simulink model "Hydraulic_Hybrid_direct"  (R2012b)
settings: Solver=ode4  StartTime=0.0  StopTime=length(speed_U)-1  FixedStep=t_samp_d  RelTol=1e-3
values from neighbouring files (symbols this model uses):
  Af = param_Af(i)    [parametric_analysis.m]    (also in settings.m = 2)
  alpha = 14.7    [settings.m]
  Cd = param_Cd(i)    [parametric_analysis.m]    (also in settings.m = 0.3)
  CHARGE_p = 0.7    [settings.m]
  eps_p = param_eps_p(i)    [parametric_analysis.m]    (also in settings.m = 3)
  eta_mech = param_eta_mech(i)    [parametric_analysis.m]    (also in settings.m = 0.8)
  f = param_f(i)    [parametric_analysis.m]    (also in settings.m = 0.015)
  gear_ratios = param_gear_ratios(i,:)    [parametric_analysis.m]    (also in settings.m = [3.6 2.1 1.4 1 0.8])
  k = 1.4    [settings.m]
  Kd = param_Kd(i)    [parametric_analysis.m]    (also in settings.m = 0.1)
  m = param_m(i)    [parametric_analysis.m]    (also in settings.m = 1200)
  n_ICE_etamax = param_n_ICE_etamax(i)    [parametric_analysis.m]    (also in settings.m = 2500)
  p_ACC_0 = param_p_ACC_0(i)    [parametric_analysis.m]    (also in settings.m = 24000000)
  p_ACC_MAX = param_p_ACC_MAX(i)    [parametric_analysis.m]    (also in settings.m = 35000000)
  p_ACC_min = param_p_ACC_min(i)    [parametric_analysis.m]    (also in settings.m = 13000000)
  p_SERB_0 = param_p_SERB_0(i)    [parametric_analysis.m]    (also in settings.m = 760000)
  p_SERB_MAX = param_p_SERB_MAX(i)    [parametric_analysis.m]    (also in settings.m = 1800000)
  p_SERB_min = param_p_SERB_min(i)    [parametric_analysis.m]    (also in settings.m = 600000)
  r_ROT = param_r_ROT(i)    [parametric_analysis.m]    (also in settings.m = 0.26)
  rho_air = 1.2    [settings.m]
  rho_fuel = 720    [settings.m]
  slope = [0 0 0 0 0 0 0 0 0 0 0 0 ... (1370 elements, 1370x1)]    [cycles.mat]
  speed_H = [0 0 0 3.22 7.889 13.041 18.193 23.345 27.853 31.556 35.098 38.64 ... (1370 elements, 1370x1)]    [cycles.mat]
  speed_U = [0 0 0 0 0 0 0 0 0 0 0 0 ... (1370 elements, 1370x1)]    [cycles.mat]
  T_brake_MAX = 200    [settings.m]
  T_n_MAX = param_T_n_MAX(i)    [parametric_analysis.m]    (also in settings.m = 60)
  T_n_min = param_T_n_min(i)    [parametric_analysis.m]    (also in settings.m = 40)
  t_react = param_t_react(i)    [parametric_analysis.m]    (also in settings.m = 0.1)
  t_samp = 1    [settings.m]
  t_samp_d = 1/5    (= 0.2)    [settings.m]
  tau = param_tau(i)    [parametric_analysis.m]    (also in settings.m = 0.1)
  torque_curve = param_torque_curve(i,:)    [parametric_analysis.m]    (also in settings.m = [n_ICE_min;(T_MAX-T_n_min)/(n_TM_min-n_ICE_min);n_TM_min;T_M)
  V_ACC_0 = param_V_ACC_0(i)    [parametric_analysis.m]    (also in settings.m = 0.0323)
  V_ICE = param_V_ICE(i)    [parametric_analysis.m]    (also in settings.m = 0.0014)
  V_PM = 45*10^(-6)    (= 4.5e-05)    [settings.m]
  V_SERB_0 = param_V_SERB_0(i)    [parametric_analysis.m]    (also in settings.m = 0.0423)
  wind_speed = [0 0 0 0 0 0 0 0 0 0 0 0 ... (1370 elements, 1370x1)]    [cycles.mat]
settings Model: Creator=MEGA  LastModifiedBy=MEGA

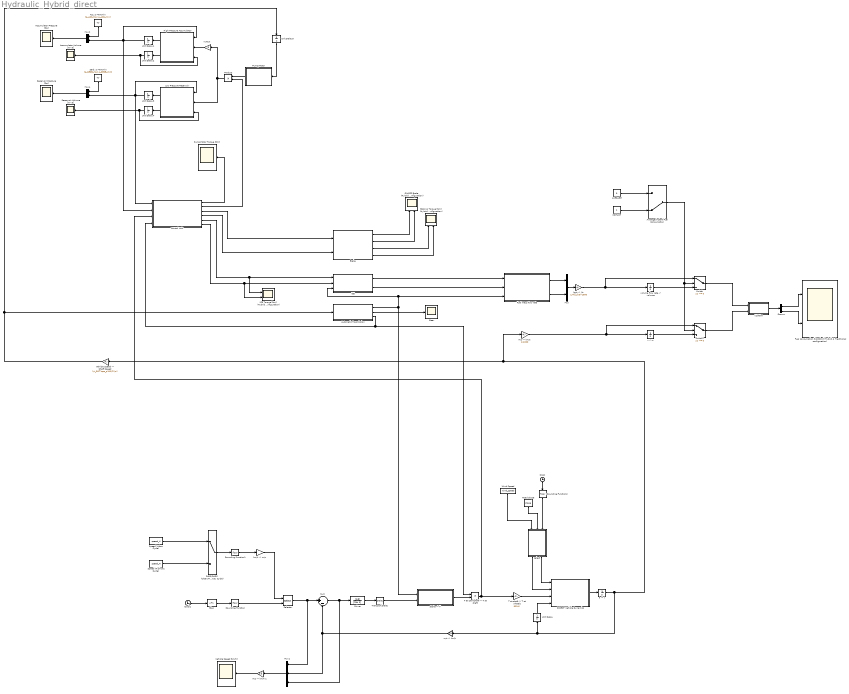
== system Hydraulic_Hybrid_direct ==
  AVERAGE : Constant  Value=0  SampleTime=t_samp_d
  Acc. p MAX/min : Constant  Value=[p_ACC_MAX p_ACC_min]  SampleTime=t_samp_d
  Accumulator Pressure [Pa] : Scope
      settings: SaveName=accum_press  SampleInput=on  SampleTime=t_samp_d
  Accumulator Volume [m^3] : Scope
      settings: SaveName=accum_vol  SampleInput=on  SampleTime=t_samp_d
  Automatic Trasmission : MATLAB Function  TreatAsAtomicUnit=on  SystemSampleTime=t_samp_d
  Average/Instant Fuel Consumption : ManualSwitch  CurrentSetting=0  SampleTime=t_samp_d
  Bias : Bias  Bias=1
  Brake : MATLAB Function  TreatAsAtomicUnit=on  SystemSampleTime=t_samp_d
  Braking Torque [Nm] (Hybrid & Traditional Configuration) : Scope  NumInputPorts=2
      settings: YMin=-5~-5  YMax=5~5  SaveName=brake_torque  DataFormat=Structure  SampleInput=on  SampleTime=t_samp_d
  Clock : Clock
  Clock1 : Clock
  Control Unit : MATLAB Function  TreatAsAtomicUnit=on  SystemSampleTime=t_samp_d
  DIRECT Vehicle Dynamics : MATLAB Function  TreatAsAtomicUnit=on  SystemSampleTime=t_samp_d
  Demux : Demux  Outputs=2
  Driver : TransferFcn  Numerator=[Kd]  Denominator=[tau 1]
  FUDS/FHDS (Urban/Highway Cycle) : ManualSwitch  SampleTime=t_samp_d
  Fuel consumption [l/100km] (Hybrid & Traditional configuration) : Scope  NumInputPorts=2
      settings: YMin=0.485~5.57  YMax=0.56~5.77  SaveName=fuel_consumption  DataFormat=Structure  SampleInput=on  SampleTime=t_samp_d
  Fuel mass flow rate : MATLAB Function  TreatAsAtomicUnit=on  SystemSampleTime=t_samp_d
  Gear : Scope
      settings: YMin=0.95  YMax=1.05  SaveName=gear  SampleInput=on  SampleTime=t_samp_d
  High Pressure Accumulator : MATLAB Function  TreatAsAtomicUnit=on  SystemSampleTime=t_samp_d
  ICE : MATLAB Function  TreatAsAtomicUnit=on  SystemSampleTime=t_samp_d
  ICE Torque [Nm] (Hybrid & Traditional Configuration) : Scope  NumInputPorts=2
      settings: YMin=-5~-5  YMax=5~5  SaveName=ICE_torque  DataFormat=Structure  SampleInput=on  SampleTime=t_samp_d
  INSTANT : Constant  SampleTime=t_samp_d
  In/Out : Gain  Gain=-1  SampleTime=t_samp_d
  Low Pressure Reservoir : MATLAB Function  TreatAsAtomicUnit=on  SystemSampleTime=t_samp_d
  Mux : Mux  Inputs=2
  Mux1 : Mux  Inputs=3
  Mux2 : Mux  Inputs=2
  Mux4 : Mux  Inputs=2
  ON/OFF Brake (Hybrid & Traditional Configuration) : Scope  NumInputPorts=2
      settings: ShowLegends=on  YMin=-5~-5  YMax=5~5  SampleInput=on  SampleTime=t_samp_d
  Product : Product  SampleTime=t_samp_d  RndMeth=Zero
  Pump/Motor : MATLAB Function  TreatAsAtomicUnit=on  SystemSampleTime=t_samp_d
  Pump/Motor Torque [Nm] : Scope
      settings: YMin=0  YMax=42.5  SaveName=hyd_torque  SampleInput=on  SampleTime=t_samp_d
  Reservoir Pressure [Pa] : Scope
      settings: SaveName=serb_press  SampleInput=on  SampleTime=t_samp_d
  Reservoir Volume [m^3] : Scope
      settings: SaveName=serb_vol  SampleInput=on  SampleTime=t_samp_d
  Road Slope : Constant  Value=slope  SampleTime=t_samp_d
  Rounding Function : Rounding  SampleTime=t_samp_d
  Rounding Function1 : Rounding  SampleTime=t_samp_d
  Rounding Function2 : Rounding  SampleTime=t_samp_d
  Selector : Selector  InputPortWidth=1370  SampleTime=t_samp_d  IndexOptions=Index vector (port)  Indices=[1 3]  OutputSizes=1
  Serb. p MAX/min : Constant  Value=[p_SERB_MAX p_SERB_min]  SampleTime=t_samp_d
  Speed (Highway Cycle) : Constant  Value=speed_H  SampleTime=t_samp_d
  Speed (Urban Cycle) : Constant  Value=speed_U  SampleTime=t_samp_d
  Sum : Sum  Inputs=|+-  SampleTime=t_samp_d
  Switch : Switch  Criteria=u2 ~= 0  SampleTime=t_samp_d
  Switch1 : Switch  Criteria=u2 ~= 0  SampleTime=t_samp_d
  "T at crankshaft -> T at shaft" : Product  SampleTime=t_samp_d  RndMeth=Zero
  "T at shaft -> T at wheels" : Gain  Gain=eps_p  SampleTime=t_samp_d
  Transport Delay : TransportDelay  DelayTime=t_react
  Unit Delay : UnitDelay  SampleTime=t_samp_d
  Unit Delay1 : UnitDelay  InitialCondition=p_ACC_0  SampleTime=t_samp_d
  Unit Delay2 : UnitDelay  InitialCondition=V_ACC_0  SampleTime=t_samp_d
  Unit Delay3 : UnitDelay  InitialCondition=p_SERB_0  SampleTime=t_samp_d
  Unit Delay4 : UnitDelay  InitialCondition=V_SERB_0  SampleTime=t_samp_d
  Unit Delay5 : UnitDelay  SampleTime=t_samp_d
  "Vehicle Speed -> Shaft Speed" : Gain  Gain=1/r_ROT*eps_p*60/(2*pi)  SampleTime=t_samp_d
  Vehicle Speed [km/h] : Scope
      settings: TimeRange=1369  YMin=-3  YMax=16  SaveName=vehicle_speed  DataFormat=Structure  SampleInput=on  SampleTime=t_samp_d
  Wind Speed : Constant  Value=wind_speed  SampleTime=t_samp_d
  "a -> v" : Integrator
  "kg/s -> l/s" : Gain  Gain=1/rho_fuel*1000  SampleTime=t_samp_d
  "km/h -> m/s" : Gain  Gain=1/3.6  SampleTime=t_samp_d
  l/100km : MATLAB Function  TreatAsAtomicUnit=on  SystemSampleTime=t_samp_d
  "m/s -> km/h" : Gain  Gain=3.6  SampleTime=t_samp_d
  "m/s -> km/h 1" : Gain  Gain=3.6  SampleTime=t_samp_d
  "m/s -> km/s" : Gain  Gain=1/1000  SampleTime=t_samp_d
  select : MATLAB Function  TreatAsAtomicUnit=on  SystemSampleTime=t_samp_d
  "stroke -> T" : MATLAB Function  TreatAsAtomicUnit=on  SystemSampleTime=t_samp_d
  "v -> s" : Integrator
  "volume flow rate -> volume" : Integrator
  wires:
  Low Pressure Reservoir/1(p_serb_i) -> Unit Delay3/1
  Product/1 -> Low Pressure Reservoir/2(Q), In/Out/1
  Control Unit/2(sign) -> Product/2
  Control Unit/1(T_PM) -> Pump/Motor Torque [Nm]/1
  Control Unit/5(T_ICE_H) -> ICE Torque [Nm] (Hybrid & Traditional Configuration)/1, ICE/1(T_ICE_H)
  Automatic Trasmission/2(gear) -> Gear/1
  Fuel mass flow rate/1(mpf_H) -> Mux/1
  Fuel mass flow rate/2(mpf_NH) -> Mux/2
  Mux/1 -> "kg/s -> l/s"/1
  "volume flow rate -> volume"/1 -> Switch/3
  Speed (Urban Cycle)/1 -> FUDS/FHDS (Urban/Highway Cycle)/1
  Speed (Highway Cycle)/1 -> FUDS/FHDS (Urban/Highway Cycle)/2
  Control Unit/3(T_BRAKE_H) -> Brake/1(T_BRAKE_H_i)
  Road Slope/1 -> select/2(slope)
  Wind Speed/1 -> select/1(wind_speed)
  Unit Delay1/1 -> High Pressure Accumulator/1(p_acc_h), Mux2/2, Control Unit/2(p_acc)
  Unit Delay3/1 -> Control Unit/1(p_serb), Mux4/2, Low Pressure Reservoir/1(p_serb_h)
  Low Pressure Reservoir/2(V_serb_i) -> Unit Delay4/1
  ICE/1(th_H) -> Fuel mass flow rate/1(th_H)
  ICE/2(th_NH) -> Fuel mass flow rate/2(th_NH)
  Pump/Motor/1(Q) -> Product/1
  High Pressure Accumulator/2(V_acc_i) -> Unit Delay2/1
  In/Out/1 -> High Pressure Accumulator/2(Q)
  Control Unit/6(T_ICE_NH) -> ICE Torque [Nm] (Hybrid & Traditional Configuration)/2, ICE/2(T_ICE_NH)
  High Pressure Accumulator/1(p_acc_i) -> Unit Delay1/1
  Clock/1 -> Rounding Function2/1
  Mux2/1 -> Accumulator Pressure [Pa]/1
  Acc. p MAX/min/1 -> Mux2/1
  Serb. p MAX/min/1 -> Mux4/1
  Unit Delay5/1 -> Pump/Motor/1(n)
  Unit Delay2/1 -> High Pressure Accumulator/3(V_acc_h), Accumulator Volume [m^3]/1
  Unit Delay4/1 -> Low Pressure Reservoir/3(V_serb_h), Reservoir Volume [m^3]/1
  FUDS/FHDS (Urban/Highway Cycle)/1 -> Rounding Function1/1
  Brake/4(T_BRAKE_NH_o) -> Braking Torque [Nm] (Hybrid & Traditional Configuration)/2
  Brake/2(on_off_NH) -> ON/OFF Brake (Hybrid & Traditional Configuration)/2
  Brake/3(T_BRAKE_H_o) -> Braking Torque [Nm] (Hybrid & Traditional Configuration)/1
  Brake/1(on_off_H) -> ON/OFF Brake (Hybrid & Traditional Configuration)/1
  AVERAGE/1 -> Average/Instant Fuel Consumption/1
  INSTANT/1 -> Average/Instant Fuel Consumption/2
  "v -> s"/1 -> Switch1/3
  "kg/s -> l/s"/1 -> "volume flow rate -> volume"/1, Switch/1
  Average/Instant Fuel Consumption/1 -> Switch1/2, Switch/2
  Switch/1 -> l/100km/1(l)
  Switch1/1 -> l/100km/2(km)
  Mux4/1 -> Reservoir Pressure [Pa]/1
  l/100km/1(c) -> Demux/1
  Demux/1 -> Fuel consumption [l/100km] (Hybrid & Traditional configuration)/1
  Demux/2 -> Fuel consumption [l/100km] (Hybrid & Traditional configuration)/2
  Sum/1 -> Mux1/3, Driver/1
  DIRECT Vehicle Dynamics/1(a) -> "a -> v"/1
  "m/s -> km/s"/1 -> Switch1/1, "v -> s"/1
  "Vehicle Speed -> Shaft Speed"/1 -> Automatic Trasmission/1(n_shaft), Unit Delay5/1
  Automatic Trasmission/1(n_ICE) -> ICE/3(n), Fuel mass flow rate/3(n_ICE), "stroke -> T"/1(n_ICE)
  Control Unit/4(T_BRAKE_NH) -> Brake/2(T_BRAKE_NH_i)
  select/1(v_w_i) -> DIRECT Vehicle Dynamics/2(v_w)
  select/2(slope_i) -> DIRECT Vehicle Dynamics/1(slope)
  Automatic Trasmission/3(eps_g) -> Control Unit/4(eps_g), "T at crankshaft -> T at shaft"/1
  "stroke -> T"/1(T) -> "T at crankshaft -> T at shaft"/2
  "T at crankshaft -> T at shaft"/1 -> "T at shaft -> T at wheels"/1, Control Unit/3(T)
  "km/h -> m/s"/1 -> Selector/1
  Clock1/1 -> Bias/1
  "a -> v"/1 -> Unit Delay/1, "m/s -> km/h"/1, "m/s -> km/s"/1, "Vehicle Speed -> Shaft Speed"/1
  Selector/1 -> Mux1/1, Sum/1
  Bias/1 -> Rounding Function/1
  Driver/1 -> Transport Delay/1
  "T at shaft -> T at wheels"/1 -> DIRECT Vehicle Dynamics/3(T)
  Mux1/1 -> "m/s -> km/h 1"/1
  Rounding Function/1 -> Selector/2
  Rounding Function1/1 -> "km/h -> m/s"/1
  Rounding Function2/1 -> select/3(t)
  Unit Delay/1 -> DIRECT Vehicle Dynamics/4(v)
  Transport Delay/1 -> "stroke -> T"/2(stroke)
  "m/s -> km/h"/1 -> Sum/2, Mux1/2
  "m/s -> km/h 1"/1 -> Vehicle Speed [km/h]/1

== matlab function Hydraulic_Hybrid_direct/Control Unit ==
  data: T_PM output; p_serb input; p_acc input; T input; eps_g input; sign output; T_BRAKE_H output; T_BRAKE_NH output; T_ICE_H output; T_ICE_NH output; p_ACC_MAX parameter; p_ACC_min parameter; p_SERB_MAX parameter; p_SERB_min parameter; CHARGE_p parameter; V_PM parameter; eps parameter
function [T_PM,sign,T_BRAKE_H,T_BRAKE_NH,T_ICE_H,T_ICE_NH]=control_unit(p_serb,p_acc,T,eps_g,p_ACC_MAX, p_ACC_min, p_SERB_MAX, p_SERB_min, CHARGE_p, V_PM, eps)

% Unità di controllo.
% A partire dai parametri in ingresso (pressioni nell'accumulatore
% e nel serbatoio, e coppia richiesta dal ciclo), gestisce l'
% erogazione/sottrazione della potenza dividendola tra
% componenti meccanici (ICE e freni) ed idraulici (pompa/turbina).

sign=0;
T_BRAKE_H=0;
T_BRAKE_NH=0;
T_ICE_H=0;
T_ICE_NH=0;
T_PM=0;

acc_full=0;
serb_full=0;
acc_empty=0;
serb_empty=0;

%Dp=abs(p_acc-p_serb);

if p_acc/p_ACC_MAX>CHARGE_p
    
    acc_full=1;
    
end

if p_serb/p_SERB_MAX>CHARGE_p
    
    serb_full=1;
    
end

if p_acc/p_ACC_min<1/CHARGE_p
    
    acc_empty=1;
    
end

if p_serb/p_SERB_min<1/CHARGE_p
    
    serb_empty=1;
    
end

if T<=0
    
    T_BRAKE_NH=T*eps;
    
    if ~acc_full && ~serb_empty
        
        sign=-1;
        
        T_PM=T;%-V_PM*Dp;
        
    else
        
        T_BRAKE_H=T*eps;
        
    end
    
else
    
    T_ICE_NH=T/eps_g;
    
    if ~serb_full && ~acc_empty
        
        sign=1;
        
        T_PM=T;%=V_PM*Dp;
        
    else
        
        T_ICE_H=T/eps_g;
        
    end
    
end


end

== matlab function Hydraulic_Hybrid_direct/stroke -> T ==
  data: n_ICE input; stroke input; T_brake_MAX parameter; T output; torque_curve parameter; T_n_min parameter; T_n_MAX parameter
function T=stroke_to_torque(n_ICE,stroke, T_brake_MAX, torque_curve, T_n_min, T_n_MAX)

% La funzione traduce in termini di coppia l'angolo di
% acceleratore, uscita del pilota.

n_min=torque_curve(1);
slope1=torque_curve(2);
n_TM_min=torque_curve(3);
T_MAX=torque_curve(4);
n_TM_MAX=torque_curve(5);
slope2=abs(torque_curve(6));
n_MAX=torque_curve(7);

if stroke<0
    
    T=stroke*T_brake_MAX;
    
else
    
    if n_ICE<=n_min
        
        T=T_n_min;
        
    elseif n_ICE>=n_MAX
        
        T=T_n_MAX;
        
    else
        
        if n_ICE<n_TM_min
            
            T_MAX_n=T_MAX-((n_TM_min-n_ICE)*slope1);
            
        elseif n_ICE>n_TM_MAX
            
            T_MAX_n=T_MAX-((n_ICE-n_TM_MAX)*slope2);
            
        else
            
            T_MAX_n=T_MAX;
            
        end
        
        T=stroke*T_MAX_n;
        
    end
    
end


end

== matlab function Hydraulic_Hybrid_direct/High Pressure Accumulator ==
  data: p_acc_h input; Q input; p_acc_i output; V_acc_h input; V_acc_i output; k parameter; t_samp parameter
function [p_acc_i,V_acc_i]=hyd_accserb(p_acc_h,Q,V_acc_h, k, t_samp)

% Accumulatore.
% Calcola pressione e volume alla fine di un periodo di
% campionamento in cui evolve una portata Q.

p_acc_i=p_acc_h*(1/(1-(Q*t_samp)/V_acc_h))^k;

V_acc_i=(p_acc_h/p_acc_i)^(1/k)*V_acc_h;%=V_acc_h+Q*t_samp;


end

== matlab function Hydraulic_Hybrid_direct/Low Pressure Reservoir ==
  data: p_serb_h input; Q input; p_serb_i output; V_serb_h input; V_serb_i output; k parameter; t_samp parameter
function [p_serb_i,V_serb_i]=hyd_accserb(p_serb_h,Q,V_serb_h, k, t_samp)

% Serbatoio.
% Calcola pressione e volume alla fine di un periodo di
% campionamento in cui evolve una portata Q.

p_serb_i=p_serb_h*(1/(1-(Q*t_samp)/V_serb_h))^k;

V_serb_i=(p_serb_h/p_serb_i)^(1/k)*V_serb_h;%=V_serb_h+Q*t_samp;


end

== matlab function Hydraulic_Hybrid_direct/Pump//Motor ==
  data: n input; Q output; V_PM parameter
function Q=pump_motor(n, V_PM)

% Pompa/motore.
% A partire dalla velocità di rotazione dell'albero
% dell'unità idraulica, calcola la portata che evolve
% durante il periodo di campionamento.

Q=V_PM*n*2*pi/60;


end

== matlab function Hydraulic_Hybrid_direct/Brake ==
  data: on_off_H output; T_BRAKE_H_i input; on_off_NH output; T_BRAKE_NH_i input; T_BRAKE_H_o output; T_BRAKE_NH_o output
function [on_off_H,on_off_NH,T_BRAKE_H_o,T_BRAKE_NH_o]=brake(T_BRAKE_H_i,T_BRAKE_NH_i)

% Freni.
% La funzione (in realtà è quasi solo un'assegnazione) ci ridà
% il valore della coppia frenante con in aggiunta il segnale
% on_off che ci dice (quasi solo a scopo informativo)
% quando si attivano i freni, sia per la configurazione
% tradizionale che per quella ibrida.

on_off_H=0;
on_off_NH=0;

if T_BRAKE_H_i~=0
    
    on_off_H=1;
    
end

T_BRAKE_H_o=T_BRAKE_H_i;

if T_BRAKE_NH_i~=0
    
    on_off_NH=1;
    
end

T_BRAKE_NH_o=T_BRAKE_NH_i;


end

== matlab function Hydraulic_Hybrid_direct/ICE ==
  data: T_ICE_H input; th_H output; T_ICE_NH input; th_NH output; n input; torque_curve parameter
function [th_H,th_NH]=ICE(T_ICE_H,T_ICE_NH,n, torque_curve)

% Motore a combustione interna.
% Calcola la posizione della farfalla in funzione della
% coppia richiesta, anche per configurazione non ibrida.
% torque_curve=[pendenza del primo tratto,abs(pendenza del secondo tratto),
% coppia massima, num giri che divide il primo e il secondo tratto,
% num giri che divide il secondo e il terzo tratto,];

n_min=torque_curve(1);
slope1=torque_curve(2);
n_TM_min=torque_curve(3);
T_MAX=torque_curve(4);
n_TM_MAX=torque_curve(5);
slope2=abs(torque_curve(6));
n_MAX=torque_curve(7);

if n<=n_min
    
    th_H=0;
    
    th_NH=0;
    
elseif n>=n_MAX
    
    th_H=90;
    
    th_NH=90;
    
else
    
    if n<n_TM_min
        
        T_MAX_n=T_MAX-((n_TM_min-n)*slope1);
        
    elseif n>n_TM_MAX
        
        T_MAX_n=T_MAX-((n-n_TM_MAX)*slope2);
        
    else
        
        T_MAX_n=T_MAX;
        
    end
    
    if T_ICE_H>=T_MAX
        
        th_H=90;
        
    else
        
        th_H=T_ICE_H/T_MAX_n*90;
        
    end
    
    if T_ICE_NH>=T_MAX
        
        th_NH=90;
        
    else
        
        th_NH=T_ICE_NH/T_MAX_n*90;
        
    end
    
end
    

end

== matlab function Hydraulic_Hybrid_direct/Automatic Trasmission ==
  data: n_shaft input; n_ICE output; gear output; n_ICE_etamax parameter; gear_ratios parameter; eps_g output
function [n_ICE,gear,eps_g]=auto_trasm(n_shaft, n_ICE_etamax, gear_ratios)

% Cambio automatico.
% Calcolo della marcia e del numero di giri effettivo
% del motore a combustione interna, a partire dalla
% velocità dell'albero di trasmissione.

G=length(gear_ratios);

n_ICE_test=zeros(G,1);

for g=1:G
    
    n_ICE_test(g)=n_shaft*gear_ratios(g);
    
end

diff_n=abs(n_ICE_test-n_ICE_etamax*ones(G,1));

[~,gear]=min(diff_n);

n_ICE=n_ICE_test(gear);

eps_g=gear_ratios(gear);


end

== matlab function Hydraulic_Hybrid_direct/Fuel mass flow rate ==
  data: th_H input; th_NH input; n_ICE input; mpf_H output; mpf_NH output; rho_air parameter; V_ICE parameter; alpha parameter; eps parameter; eta_mech parameter
function [mpf_H,mpf_NH]=fuelmassflowrate(th_H,th_NH,n_ICE, rho_air, V_ICE, alpha, eps, eta_mech)

% Portata massica di combustibile.
% Calcolo della portata di combustibile a partire dal valore
% dell'angolo della farfalla, anche anche per configurazione non ibrida.

lv_H=th_H/90;

lv_NH=th_NH/90;

mpf_H=lv_H*rho_air*V_ICE*n_ICE/(alpha*60*eps)/eta_mech;

mpf_NH=lv_NH*rho_air*V_ICE*n_ICE/(alpha*60*eps)/eta_mech;


end

== matlab function Hydraulic_Hybrid_direct/DIRECT Vehicle Dynamics ==
  data: slope input; v_w input; T input; a output; v input; rho_air parameter; Cd parameter; Af parameter; m parameter; f parameter; r_ROT parameter
function a=direct_veh_dyn(slope,v_w,T,v, rho_air, Cd, Af, m, f, r_ROT)

% La funzione rappresenta la dinamica (diretta) del sistema autoveicolo
% da controllare. Essa infatti fornisce in output l'accelerazione
% leggendo in input la coppia alle ruote motrici.

g=9.81; %[m/s^2]

if v==0
    
    k=0;
    
else
    
    k=1;
    
end

a=1/m*(T/r_ROT-1/2*rho_air*Cd*Af*(v+v_w)^2-k*f*m*g*cos(slope)-m*g*sin(slope));


end

== matlab function Hydraulic_Hybrid_direct/select ==
  data: wind_speed input; v_w_i output; slope input; t input; slope_i output; t_samp parameter
function [v_w_i,slope_i]=select_i(wind_speed,slope,t, t_samp)

% La funzione seleziona il valore della velocità del vento e
% della pendenza della strada per ogni istante t_i.

i=t/t_samp;

if i<length(wind_speed)
    
    v_w_i=wind_speed(i+1);
    
    slope_i=slope(i+1);
    
else
    
    v_w_i=0;
    
    slope_i=0;
    
end


end

== matlab function Hydraulic_Hybrid_direct/l//100km ==
  data: l input; c output; km input
function c=divide(l,km)

% La funzione divide calcola il valore di consumo in l/100km, prevenendo
% una divisione per 0 al primo istante di simulazione, quando i km
% percorsi sono ancora 0.

if km==0
    
    c=[0;0];
    
else
    
    c=(l/km)*100;
    
end


end
